simulink model "LPDs_single_agent_tech"  (R2023b)
settings: Solver=VariableStepAuto  StartTime=0.0  StopTime=24  FixedStep=0.005  RelTol=1e-6
undefined symbols (not defined in the file): battery_capacity_state_lower_limit, battery_capacity_state_upper_limit, battery_charge_power_state_lower_limit, battery_charge_power_state_upper_limit, battery_discharge_power_state_lower_limit, battery_discharge_power_state_upper_limit, battery_initial_capacity, battery_SOC_state_lower_limit, battery_SOC_state_upper_limit, EV_load_priority_factor, EV_load_rating, EV_load_state_lower_limit, EV_load_state_upper_limit, micro_grid_controller_power_state_lower_limit, micro_grid_controller_power_state_upper_limit, nano_grid_controller_power_rating, nano_grid_controller_power_state_lower_limit, nano_grid_controller_power_state_upper_limit, PV_power_rating, PV_power_state_lower_limit, PV_power_state_upper_limit, static_load_priority_factor, static_load_rating, static_load_state_lower_limit, static_load_state_upper_limit, sum_power_threshold_lower_limit, sum_power_threshold_upper_limit, TCL_load_priority_factor, TCL_load_rating, TCL_load_state_lower_limit, TCL_load_state_upper_limit, Wind_power_rating, Wind_power_state_lower_limit, Wind_power_state_upper_limit
libraries: spsStairGeneratorLib x13, simulink x7, slpidlib x2, rllib x2
(part 1 of 4)
settings Model: SimulationMode=accelerator  Creator=zainn  LastModifiedBy=zainn
settings DebuggingCC: StringTruncationChecking=warning  SignalRangeChecking=warning  SFUnexpectedBacktrackingDiag=warning  SFNoUnconditionalDefaultTransitionDiag=warning  SFOutputUsedAsStateInMooreChartDiag=warning  UnderSpecifiedDimensionMsg=warning

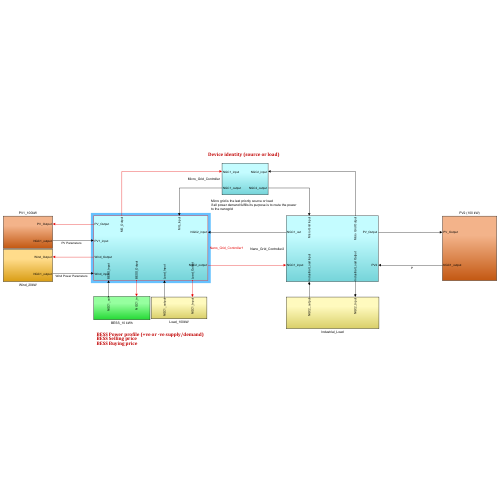
[thumbnail: Simulink's stored preview of the top-level diagram]
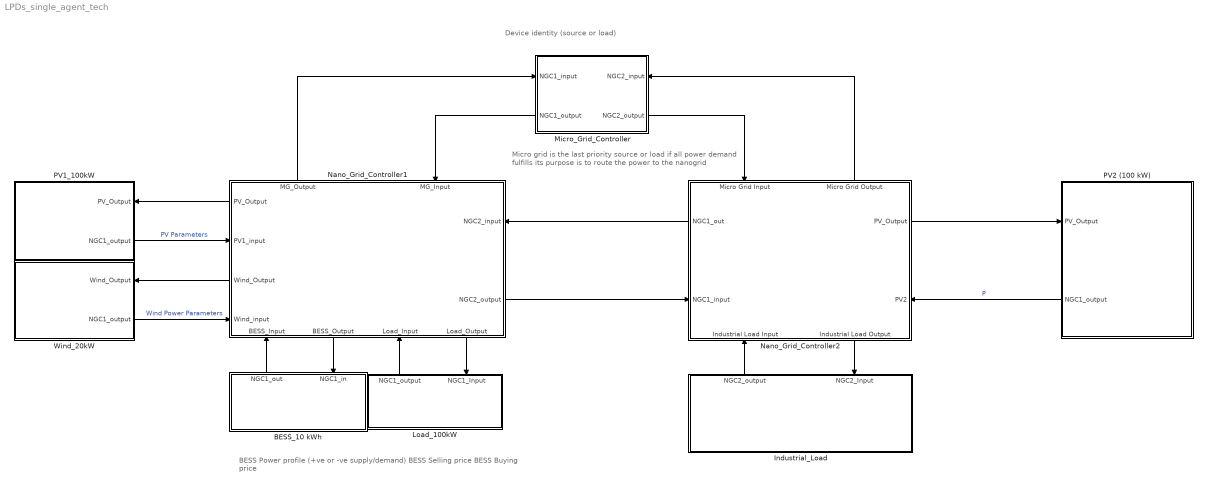
== system LPDs_single_agent_tech ==
  note: Micro grid is the last priority source or load
      | if all power demand fulfills its purpose is to route the power
      | to the nanogrid
  note: BESS Power profile (+ve or -ve supply/demand)
      | BESS Selling price
      | BESS Buying price
  note: Device identity (source or load)
  BESS_10 kWh : Subsystem
      settings: PortSchema="{\"entries\":[{\"content\":{\"sides\":[{\"content\":{},\"type\":\"ConnectorPlacement.EquallySpacedRectSide\",\"uuid\":\"e3de0fdd-9ded-4814-8a28-7acef72e72b2\"},{\"content\":{\"side\":\"RIGHT\"},\"type\":\"ConnectorPlacement.EquallySpacedRectSide\",\"uuid\":\"1903caed-e2e3-4057-bbe0-c9df58686077\"},{\"content\":{\"connectorIds\":[\"Out1\",\"In1\"],\"side\":\"TOP\"},\"type\":\"ConnectorPlacement.EquallySpacedRectSide\",\"uuid\":\"fc459ed4-5de3-49f1-9363-536f2a8ba7f9\"}]},\"type\":\"ConnectorPlacement.EquallySpacedConnector\",\"uuid\":\"56317309-16e5-499a-8db1-424ce7aac051\"}],\"packageUris\":[\"http://schema.mathworks.com/mf0/Connector/R2020b\"],\"version\":\"1.0\"}"
  Industrial_Load : Subsystem
      settings: PortSchema="{\"entries\":[{\"content\":{\"sides\":[{\"content\":{},\"type\":\"ConnectorPlacement.EquallySpacedRectSide\",\"uuid\":\"0da6eb76-3d1f-4d22-baf5-7ff34ff7c574\"},{\"content\":{\"side\":\"RIGHT\"},\"type\":\"ConnectorPlacement.EquallySpacedRectSide\",\"uuid\":\"44fb93d7-0974-45a7-8380-f34e52fb491c\"},{\"content\":{\"connectorIds\":[\"Out1\",\"In1\"],\"side\":\"TOP\"},\"type\":\"ConnectorPlacement.EquallySpacedRectSide\",\"uuid\":\"a517cdf0-6705-4d20-a9eb-30a7259bd3ad\"}]},\"type\":\"ConnectorPlacement.EquallySpacedConnector\",\"uuid\":\"0aa8bbf3-fb90-49da-9b11-c21fdfaeaa79\"}],\"packageUris\":[\"http://schema.mathworks.com/mf0/Connector/R2020b\"],\"version\":\"1.0\"}"
  Load_100kW : Subsystem
      settings: PortSchema="{\"entries\":[{\"content\":{\"sides\":[{\"content\":{},\"type\":\"ConnectorPlacement.EquallySpacedRectSide\",\"uuid\":\"0da6eb76-3d1f-4d22-baf5-7ff34ff7c574\"},{\"content\":{\"side\":\"RIGHT\"},\"type\":\"ConnectorPlacement.EquallySpacedRectSide\",\"uuid\":\"44fb93d7-0974-45a7-8380-f34e52fb491c\"},{\"content\":{\"connectorIds\":[\"Out1\",\"In1\"],\"side\":\"TOP\"},\"type\":\"ConnectorPlacement.EquallySpacedRectSide\",\"uuid\":\"a517cdf0-6705-4d20-a9eb-30a7259bd3ad\"}]},\"type\":\"ConnectorPlacement.EquallySpacedConnector\",\"uuid\":\"0aa8bbf3-fb90-49da-9b11-c21fdfaeaa79\"}],\"packageUris\":[\"http://schema.mathworks.com/mf0/Connector/R2020b\"],\"version\":\"1.0\"}"
  Micro_Grid_Controller : Subsystem
      settings: PortSchema="{\"entries\":[{\"content\":{\"sides\":[{\"content\":{\"connectorIds\":[\"In1\",\"Out2\"]},\"type\":\"ConnectorPlacement.EquallySpacedRectSide\",\"uuid\":\"e3de0fdd-9ded-4814-8a28-7acef72e72b2\"},{\"content\":{\"connectorIds\":[\"In2\",\"Out1\"],\"side\":\"RIGHT\"},\"type\":\"ConnectorPlacement.EquallySpacedRectSide\",\"uuid\":\"1903caed-e2e3-4057-bbe0-c9df58686077\"},{\"content\":{\"side\":\"TOP\"},\"type\":\"ConnectorPlacement.EquallySpacedRectSide\",\"uuid\":\"fc459ed4-5de3-49f1-9363-536f2a8ba7f9\"}]},\"type\":\"ConnectorPlacement.EquallySpacedConnector\",\"uuid\":\"56317309-16e5-499a-8db1-424ce7aac051\"}],\"packageUris\":[\"http://schema.mathworks.com/mf0/Connector/R2020b\"],\"version\":\"1.0\"}"
  Nano_Grid_Controller1 : Subsystem
      settings: PortSchema="{\"entries\":[{\"content\":{\"sides\":[{\"content\":{\"connectorIds\":[\"Out5\",\"In1\",\"Out6\",\"In2\"]},\"type\":\"ConnectorPlacement.EquallySpacedRectSide\",\"uuid\":\"e3de0fdd-9ded-4814-8a28-7acef72e72b2\"},{\"content\":{\"connectorIds\":[\"In6\",\"Out1\"],\"side\":\"RIGHT\"},\"type\":\"ConnectorPlacement.EquallySpacedRectSide\",\"uuid\":\"1903caed-e2e3-4057-bbe0-c9df58686077\"},{\"content\":{\"connectorIds\":[\"Out4\",\"In3\"],\"side\":\"TOP\"},\"type\":\"ConnectorPlacement.EquallySpacedRectSide\",\"uuid\":\"fc459ed4-5de3-49f1-9363-536f2a8ba7f9\"},{\"content\":{\"connectorIds\":[\"In4\",\"Out2\",\"In5\",\"Out3\"],\"side\":\"BOTTOM\"},\"type\":\"ConnectorPlacement.EquallySpacedRectSide\",\"uuid\":\"1c798d9e-0dca-4d49-ab65-a1e33a647ade\"}]},\"type\":\"ConnectorPlacement.EquallySpacedConnector\",\"uuid\":\"56317309-16e5-499a-8db1-424ce7aac051\"}],\"packageUris\":[\"http://schema.mathworks.com/mf0/Connector/R2020b\"],\"version\":\"1.0\"}"
  Nano_Grid_Controller2 : Subsystem
      settings: PortSchema="{\"entries\":[{\"content\":{\"sides\":[{\"content\":{\"connectorIds\":[\"Out4\",\"In1\"]},\"type\":\"ConnectorPlacement.EquallySpacedRectSide\",\"uuid\":\"e3de0fdd-9ded-4814-8a28-7acef72e72b2\"},{\"content\":{\"connectorIds\":[\"Out1\",\"In4\"],\"side\":\"RIGHT\"},\"type\":\"ConnectorPlacement.EquallySpacedRectSide\",\"uuid\":\"1903caed-e2e3-4057-bbe0-c9df58686077\"},{\"content\":{\"connectorIds\":[\"In2\",\"Out3\"],\"side\":\"TOP\"},\"type\":\"ConnectorPlacement.EquallySpacedRectSide\",\"uuid\":\"fc459ed4-5de3-49f1-9363-536f2a8ba7f9\"},{\"content\":{\"connectorIds\":[\"In3\",\"Out2\"],\"side\":\"BOTTOM\"},\"type\":\"ConnectorPlacement.EquallySpacedRectSide\",\"uuid\":\"1c798d9e-0dca-4d49-ab65-a1e33a647ade\"}]},\"type\":\"ConnectorPlacement.EquallySpacedConnector\",\"uuid\":\"56317309-16e5-499a-8db1-424ce7aac051\"}],\"packageUris\":[\"http://schema.mathworks.com/mf0/Connector/R2020b\"],\"version\":\"1.0\"}"
  PV1_100kW : Subsystem
      settings: PortSchema="{\"entries\":[{\"content\":{\"sides\":[{\"content\":{},\"type\":\"ConnectorPlacement.EquallySpacedRectSide\",\"uuid\":\"7032c1f9-1959-4513-a54d-b69755860499\"},{\"content\":{\"connectorIds\":[\"In1\",\"Out1\"],\"side\":\"RIGHT\"},\"type\":\"ConnectorPlacement.EquallySpacedRectSide\",\"uuid\":\"9a429717-82a2-4906-bd67-8a0098e92bc5\"},{\"content\":{\"side\":\"TOP\"},\"type\":\"ConnectorPlacement.EquallySpacedRectSide\",\"uuid\":\"42d6152d-cb5d-47c6-94e3-860cc7e00aa3\"}]},\"type\":\"ConnectorPlacement.EquallySpacedConnector\",\"uuid\":\"6009fa80-3f39-4509-b907-d8928449430c\"}],\"packageUris\":[\"http://schema.mathworks.com/mf0/Connector/R2020b\"],\"version\":\"1.0\"}"
  PV2 (100 kW) : Subsystem
      settings: PortSchema="{\"entries\":[{\"content\":{\"sides\":[{\"content\":{\"connectorIds\":[\"In1\",\"Out1\"]},\"type\":\"ConnectorPlacement.EquallySpacedRectSide\",\"uuid\":\"7032c1f9-1959-4513-a54d-b69755860499\"},{\"content\":{\"side\":\"RIGHT\"},\"type\":\"ConnectorPlacement.EquallySpacedRectSide\",\"uuid\":\"9a429717-82a2-4906-bd67-8a0098e92bc5\"},{\"content\":{\"side\":\"TOP\"},\"type\":\"ConnectorPlacement.EquallySpacedRectSide\",\"uuid\":\"42d6152d-cb5d-47c6-94e3-860cc7e00aa3\"}]},\"type\":\"ConnectorPlacement.EquallySpacedConnector\",\"uuid\":\"6009fa80-3f39-4509-b907-d8928449430c\"}],\"packageUris\":[\"http://schema.mathworks.com/mf0/Connector/R2020b\"],\"version\":\"1.0\"}"
  Wind_20kW : Subsystem
      settings: PortSchema="{\"entries\":[{\"content\":{\"sides\":[{\"content\":{},\"type\":\"ConnectorPlacement.EquallySpacedRectSide\",\"uuid\":\"03076aaf-7345-483d-8b03-661c38e681de\"},{\"content\":{\"connectorIds\":[\"In1\",\"Out1\"],\"side\":\"RIGHT\"},\"type\":\"ConnectorPlacement.EquallySpacedRectSide\",\"uuid\":\"a6a7b42d-666f-4303-b02c-0e0b4faf9970\"},{\"content\":{\"side\":\"TOP\"},\"type\":\"ConnectorPlacement.EquallySpacedRectSide\",\"uuid\":\"fc7f3343-50d1-4ad7-a11b-2a23723237ab\"}]},\"type\":\"ConnectorPlacement.EquallySpacedConnector\",\"uuid\":\"09f58893-889c-451e-84b3-0504517d028c\"}],\"packageUris\":[\"http://schema.mathworks.com/mf0/Connector/R2020b\"],\"version\":\"1.0\"}"
  wires:
  Nano_Grid_Controller2/4(NGC1_out) -> Nano_Grid_Controller1/6(NGC2_input)
  Micro_Grid_Controller/2(NGC1_output) -> Nano_Grid_Controller1/3(MG_Input)
  Nano_Grid_Controller1/2(BESS_Output) -> BESS_10 kWh/1(NGC1_in)
  PV2 (100 kW)/1(NGC1_output) -> Nano_Grid_Controller2/4(PV2)  "P"
  Wind_20kW/1(NGC1_output) -> Nano_Grid_Controller1/2(Wind_input)  "Wind Power Parameters"
  Micro_Grid_Controller/1(NGC2_output) -> Nano_Grid_Controller2/2(Micro Grid Input)
  Nano_Grid_Controller1/1(NGC2_output) -> Nano_Grid_Controller2/1(NGC1_input)
  BESS_10 kWh/1(NGC1_out) -> Nano_Grid_Controller1/4(BESS_Input)
  Nano_Grid_Controller2/3(Micro Grid Output) -> Micro_Grid_Controller/2(NGC2_input)
  Nano_Grid_Controller2/2(Industrial Load Output) -> Industrial_Load/1(NGC2_Input)
  Nano_Grid_Controller1/4(MG_Output) -> Micro_Grid_Controller/1(NGC1_input)
  PV1_100kW/1(NGC1_output) -> Nano_Grid_Controller1/1(PV1_input)  "PV Parameters"
  Nano_Grid_Controller1/3(Load_Output) -> Load_100kW/1(NGC1_Input)
  Load_100kW/1(NGC1_output) -> Nano_Grid_Controller1/5(Load_Input)
  Industrial_Load/1(NGC2_output) -> Nano_Grid_Controller2/3(Industrial Load Input)
  Nano_Grid_Controller1/5(PV_Output) -> PV1_100kW/1(PV_Output)
  Nano_Grid_Controller1/6(Wind_Output) -> Wind_20kW/1(Wind_Output)
  Nano_Grid_Controller2/1(PV_Output) -> PV2 (100 kW)/1(PV_Output)

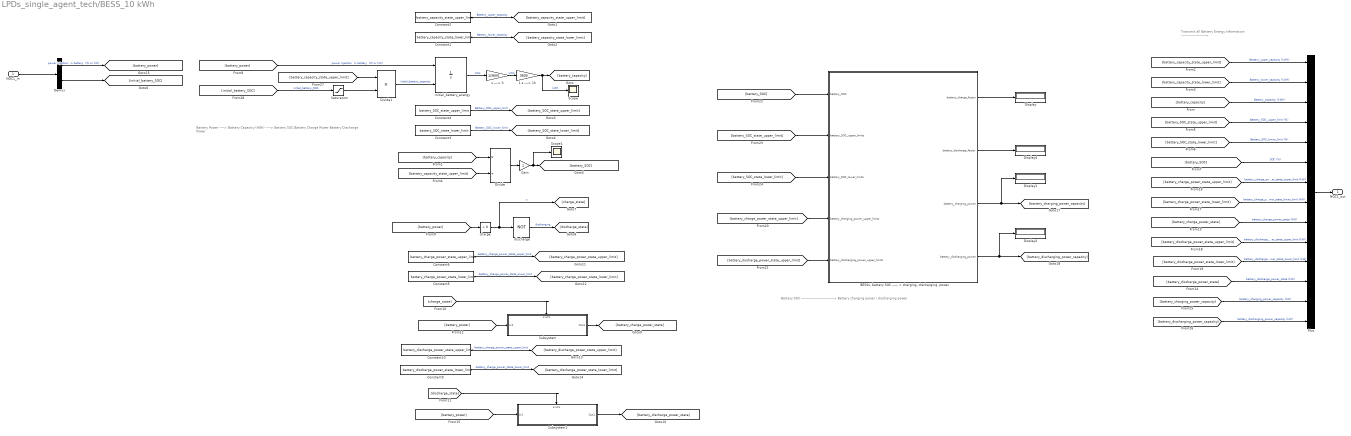
== system LPDs_single_agent_tech/BESS_10 kWh ==
  note: Transmit all Battery Energy Information
      | ------------------------->
  note: Battery Power -----> Battery Capacity (kWh) -----> Battery SOC Battery Charge Power
      | Battery Discharge Power
  note: Battery SOC ---------------------------------> Battery charging power / discharging power
  NGC1_in : Inport
  1 s ----> 1h : Gain  Gain=3600
  "BESSs, battery SOC ------ > charging, discharging. power" : Stateflow chart  TreatAsAtomicUnit=on
  Constant1 : Constant  Value=battery_capacity_state_lower_limit
  Constant10 : Constant  Value=battery_discharge_power_state_upper_limit
  Constant2 : Constant  Value=battery_capacity_state_upper_limit
  Constant3 : Constant  Value=battery_SOC_state_lower_limit
  Constant4 : Constant  Value=battery_SOC_state_upper_limit
  Constant5 : Constant  Value=battery_charge_power_state_lower_limit
  Constant6 : Constant  Value=battery_charge_power_state_upper_limit
  Constant9 : Constant  Value=battery_discharge_power_state_lower_limit
  Demux : Demux  Outputs=2
  Display{,1..2,4} (4 alike) : Display
  Divide : Product  Inputs=*/
  Divide1 : Product  Inputs=**
  Gain : Gain
  Mux : Mux  Inputs=14
  Saturation : Saturate  UpperLimit=1  LowerLimit=0
  Scope : Scope
  Scope1 : Scope
  Subsystem : Subsystem
  Subsystem1 : Subsystem
  charge : simulink/Logic and Bit Operations/Compare To Zero  relop=>  OutDataTypeStr=boolean
  discharge : Logic  Operator=NOT  IconShape=distinctive  AllPortsSameDT=off  OutDataTypeStr=boolean
  initial_battery_energy : Integrator  InitialConditionSource=external  InitialCondition=battery_initial_capacity
  s ----> h : Gain  Gain=1/3600
  NGC1_out : Outport
  wires:
  Mux/1 -> NGC1_out/1
  [battery_SOC] -> Mux/6  "SOC (%)"
  [battery_capacity_state_upper_limit] -> Mux/1  "Battery_upper_capacity (kWh)"
  [battery_capacity_state_lower_limit] -> Mux/2  "Battery_lower_capacity (kWh)"
  [battery_SOC_state_upper_limit] -> Mux/4  "Battery_SOC_upper_limit (%)"
  [battery_SOC_state_lower_limit] -> Mux/5  "Battery_SOC_lower_limit (%)"
  [battery_capacity] -> Mux/3  "Battery_capacity (kWh)"
  [battery_charge_power_state_lower_limit] -> Mux/8  "battery_charge_power_state_lower_limit (kW)"
  [battery_charge_power_state] -> Mux/9  "battery_charge_power_state (kW)"
  [battery_charge_power_state_upper_limit] -> Mux/7  "battery_charge_power_state_upper_limit (kW)"
  [battery_discharge_power_state_upper_limit] -> Mux/10  "battery_discharge_power_state_upper_limit (kW)"
  [battery_discharge_power_state] -> Mux/12  "battery_discharge_power_state (kW)"
  [battery_discharge_power_state_lower_limit] -> Mux/11  "battery_discharge_power_state_lower_limit (kW)"
  [battery_power] -> initial_battery_energy/1  "power injection  in battery  (W or kW)"
  initial_battery_energy/1 -> s ----> h/1  "kWs"
  s ----> h/1 -> 1 s ----> 1h/1  "kWh"
  1 s ----> 1h/1 -> Scope/1, [battery_capacity]  "kWh"
  Constant2/1 -> [battery_capacity_state_upper_limit]  "Battery_upper_capacity"
  Constant1/1 -> [battery_capacity_state_lower_limit]  "Battery_lower_capacity"
  [battery_capacity] -> Divide/1
  [battery_capacity_state_upper_limit] -> Divide/2
  Constant4/1 -> [battery_SOC_state_upper_limit]  "Battery_SOC_upper_limit"
  Constant3/1 -> [battery_SOC_state_lower_limit]  "Battery_SOC_lower_limit"
  Divide/1 -> Gain/1
  charge/1 -> discharge/1, [charge_state]  "s"
  [battery_power] -> charge/1
  discharge/1 -> [discharge_state]  "discharging"
  [charge_state] -> Subsystem/Enable
  [battery_power] -> Subsystem/1(In1)
  [discharge_state] -> Subsystem1/Enable
  Subsystem1/1(Out1) -> [battery_discharge_power_state]
  [battery_power] -> Subsystem1/1(In1)
  Constant6/1 -> [battery_charge_power_state_upper_limit]  "battery_charge_power_state_upper_limit"
  Constant5/1 -> [battery_charge_power_state_lower_limit]  "battery_charge_power_state_lower_limit"
  Constant10/1 -> [battery_discharge_power_state_upper_limit]  "battery_charge_power_state_upper_limit"
  Constant9/1 -> [battery_discharge_power_state_lower_limit]  "battery_charge_power_state_lower_limit"
  Subsystem/1(Out1) -> [battery_charge_power_state]
  Gain/1 -> Scope1/1, [battery_SOC]
  [battery_SOC] -> "BESSs, battery SOC ------ > charging, discharging. power"/1(battery_SOC)
  [battery_charge_power_state_upper_limit] -> "BESSs, battery SOC ------ > charging, discharging. power"/4(battery_charging_power_upper_limits)
  "BESSs, battery SOC ------ > charging, discharging. power"/1(battery_charge_factor) -> Display/1
  "BESSs, battery SOC ------ > charging, discharging. power"/4(battery_discharging_power) -> [battery_discharging_power_capacity], Display2/1
  [battery_discharge_power_state_upper_limit] -> "BESSs, battery SOC ------ > charging, discharging. power"/5(battery_discharging_power_upper_limits)
  "BESSs, battery SOC ------ > charging, discharging. power"/3(battery_charging_power) -> [battery_charging_power_capacity], Display1/1
  "BESSs, battery SOC ------ > charging, discharging. power"/2(battery_discharge_factor) -> Display4/1
  [battery_SOC_state_upper_limit] -> "BESSs, battery SOC ------ > charging, discharging. power"/2(battery_SOC_upper_limits)
  [battery_SOC_state_lower_limit] -> "BESSs, battery SOC ------ > charging, discharging. power"/3(battery_SOC_lower_limits)
  [battery_charging_power_capacity] -> Mux/13  "battery_charging_power_capacity (kW)"
  [battery_discharging_power_capacity] -> Mux/14  "battery_discharging_power_capacity (kW)"
  Divide1/1 -> initial_battery_energy/2  "initial_battery_capacity"
  [battery_capacity_state_upper_limit] -> Divide1/1
  [initial_battery_SOC] -> Saturation/1  "initial_battery_SOC"
  NGC1_in/1 -> Demux/1
  Demux/1 -> [battery_power]  "power injection  in battery  (W or kW)"
  Demux/2 -> [initial_battery_SOC]
  Saturation/1 -> Divide1/2

== system LPDs_single_agent_tech/Industrial_Load ==
  note: Transmit all Load Information
      | ------------------------->
  NGC2_Input : Inport
  Constant1 : Constant  Value=static_load_state_lower_limit
  Constant2 : Constant  Value=static_load_state_upper_limit
  Constant3 : Constant  Value=TCL_load_state_lower_limit
  Constant4 : Constant  Value=TCL_load_state_upper_limit
  Constant5 : Constant  Value=EV_load_state_lower_limit
  Constant6 : Constant  Value=EV_load_state_upper_limit
  EV_Load : spsStairGeneratorLib/Stair Generator  t=[0]  e=1  Ts=0
  Mux : Mux  Inputs=9
  Static_Load : spsStairGeneratorLib/Stair Generator  t=[0]  e=1  Ts=0
  TCL_Load : spsStairGeneratorLib/Stair Generator  t=[0]  e=1  Ts=0
  NGC2_output : Outport
  wires:
  Static_Load/1 -> Mux/3  "Static_Load"
  TCL_Load/1 -> Mux/6  "TCL_Load"
  Mux/1 -> NGC2_output/1
  EV_Load/1 -> Mux/9  "EV_Load"
  Constant2/1 -> Mux/1  "static_load_upper_capacity"
  Constant1/1 -> Mux/2  "static_load_lower_capacity"
  Constant3/1 -> Mux/5  "TCL_load_lower_capacity"
  Constant4/1 -> Mux/4  "TCL_load_upper_capacity"
  Constant5/1 -> Mux/8  "EV_load_lower_capacity"
  Constant6/1 -> Mux/7  "EV_load_upper_capacity"

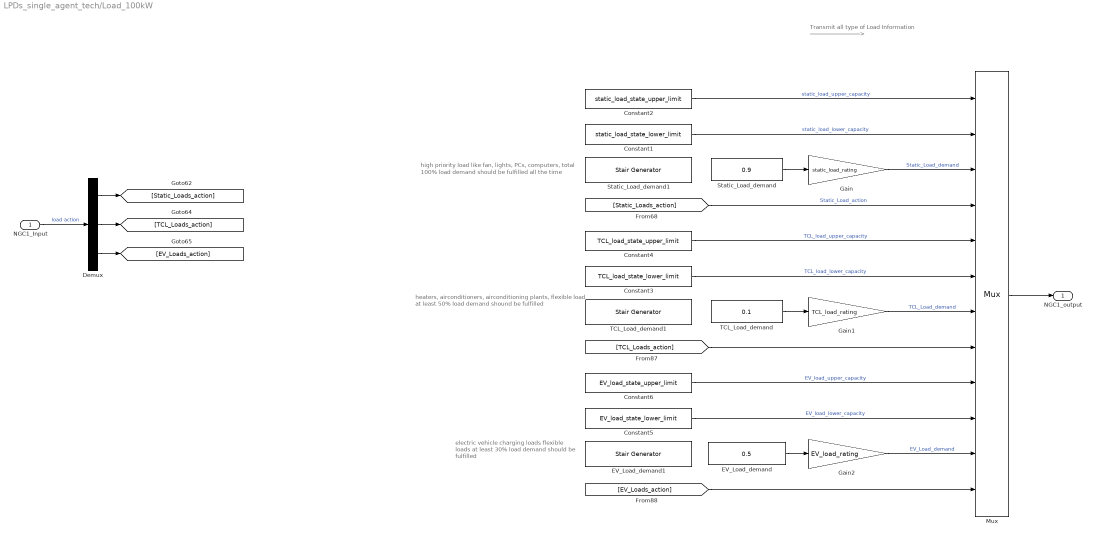
== system LPDs_single_agent_tech/Load_100kW ==
  note: high priority load like fan, lights, PCs, computers,
      | total 100% load demand should be fulfilled all the time
  note: Transmit all type of Load Information
      | ------------------------->
  note: heaters, airconditioners, airconditioning plants,
      | flexible load at least 50% load demand shound be fulfilled
  note: electric vehicle charging loads
      | flexible loads at least 30% load demand
      | should be fulfilled
  NGC1_Input : Inport
  Constant1 : Constant  Value=static_load_state_lower_limit
  Constant2 : Constant  Value=static_load_state_upper_limit
  Constant3 : Constant  Value=TCL_load_state_lower_limit
  Constant4 : Constant  Value=TCL_load_state_upper_limit
  Constant5 : Constant  Value=EV_load_state_lower_limit
  Constant6 : Constant  Value=EV_load_state_upper_limit
  Demux : Demux  Outputs=3
  EV_Load_demand : Constant  Value=0.5
  EV_Load_demand1 : spsStairGeneratorLib/Stair Generator  t=[0, 1, 2, 3, 4, 5, 6, 7, 8, 9, 10, 11, 12, 13, 14, 15, 16, 17, 18, 19, 20, 21, 22, 23]  e=[0, 0, 0, 0, 0.3, 0.3, 0.3, 0.5, 0.5, 0.5, 0.7, 0.7, 0.9, 0.9, 1, 0.8, 0.6, 0.4, 0.2, 0, 0, 0, 0, 0]  Ts=0
  Gain : Gain  Gain=static_load_rating
  Gain1 : Gain  Gain=TCL_load_rating
  Gain2 : Gain  Gain=EV_load_rating
  Mux : Mux  Inputs=12
  Static_Load_demand : Constant  Value=0.9
  Static_Load_demand1 : spsStairGeneratorLib/Stair Generator  t=[0, 1, 2, 3, 4, 5, 6, 7, 8, 9, 10, 11, 12, 13, 14, 15, 16, 17, 18, 19, 20, 21, 22, 23]  e=[0, 0.1, 0.2, 0.2, 0.3, 0.3, 0.4, 0.4, 0.5, 0.5, 0.6, 0.6, 0.7, 0.7, 0.8, 0.8, 0.9, 0.9, 1, 1, 0.9, 0.8, 0.7, 0.6]  Ts=0
  TCL_Load_demand : Constant  Value=0.1
  TCL_Load_demand1 : spsStairGeneratorLib/Stair Generator  t=[0, 1, 2, 3, 4, 5, 6, 7, 8, 9, 10, 11, 12, 13, 14, 15, 16, 17, 18, 19, 20, 21, 22, 23]  e=[0, 0, 0, 0, 0, 0, 0, 0.1, 0.3, 0.5, 0.7, 0.7, 0.8, 0.9, 1, 0.8, 0.6, 0.4, 0.2, 0, 0, 0, 0, 0]  Ts=0
  NGC1_output : Outport
  wires:
  Static_Load_demand/1 -> Gain/1
  TCL_Load_demand/1 -> Gain1/1
  Mux/1 -> NGC1_output/1
  Constant2/1 -> Mux/1  "static_load_upper_capacity"
  Constant1/1 -> Mux/2  "static_load_lower_capacity"
  Constant3/1 -> Mux/6  "TCL_load_lower_capacity"
  Constant4/1 -> Mux/5  "TCL_load_upper_capacity"
  Constant5/1 -> Mux/10  "EV_load_lower_capacity"
  Constant6/1 -> Mux/9  "EV_load_upper_capacity"
  [Static_Loads_action] -> Mux/4  "Static_Load_action"
  [TCL_Loads_action] -> Mux/8
  [EV_Loads_action] -> Mux/12
  Demux/2 -> [TCL_Loads_action]
  Demux/1 -> [Static_Loads_action]
  Demux/3 -> [EV_Loads_action]
  NGC1_Input/1 -> Demux/1  "load action"
  Gain/1 -> Mux/3  "Static_Load_demand"
  Gain1/1 -> Mux/7  "TCL_Load_demand"
  Gain2/1 -> Mux/11  "EV_Load_demand"
  EV_Load_demand/1 -> Gain2/1

== system LPDs_single_agent_tech/Micro_Grid_Controller ==
  NGC1_input : Inport
  NGC2_input : Inport  Port=2
  Constant : Constant  Value=micro_grid_controller_power_state_upper_limit
  Constant1 : Constant  Value=micro_grid_controller_power_state_lower_limit
  Gain : Gain
  Mux : Mux
  micro_grid_controller_power_state : Constant  Value=1e6
  NGC2_output : Outport
  NGC1_output : Outport  Port=2
  wires:
  Constant/1 -> Mux/1  "micro_grid_power_upper_capacity"
  micro_grid_controller_power_state/1 -> Gain/1
  Mux/1 -> NGC2_output/1, NGC1_output/1
  Constant1/1 -> Mux/2  "micro_grid_power_lower_capacity"
  Gain/1 -> Mux/3  "micro_grid_power"
  [micro_grid_controller_action] -> Mux/4
